simulink model "ibob_phased_array_2k"  (Simulink 7.0)
settings: Solver=ode45  StartTime=0.0  StopTime=70  RelTol=1e-3
undefined symbols (not defined in the file or in its folder): iBOB
libraries: xbsIndex_r4 x666, xps_library x63, beamform x4, casper_library x3
(part 2 of 6)

== system ibob_phased_array_2k/demux2 ==
  vin : Inport  OutDataType=sfix(16)  OutScaling=2^0
  in : Inport  Port=2  OutDataType=sfix(16)  OutScaling=2^0
  Counter : xbsIndex_r4/Counter  cnt_type=Free Running  cnt_to=Inf  operation=Up  start_count=0  cnt_by_val=1  arith_type=Unsigned  n_bits=1  bin_pt=0  load_pin=off  rst=off  en=on  explicit_period=off  period=1  dbl_ovrd=off  use_behavioral_HDL=off  use_rpm=on  implementation=Fabric  block_type=counter
      settings: xl_area=[0, 0, 0, 0, 0, 0, 0]
  Down Sample : xbsIndex_r4/Down Sample  sample_ratio=2  sample_phase=First Value of Frame  en=off  latency=1  dbl_ovrd=off  block_type=dsamp
      settings: xl_area=[0, 0, 0, 0, 0, 0, 0]  block_version=10.1.3
  Down Sample1 : xbsIndex_r4/Down Sample  sample_ratio=2  sample_phase="Last Value of Frame  (most efficient)"  en=off  latency=1  dbl_ovrd=off  block_type=dsamp
      settings: xl_area=[0, 0, 0, 0, 0, 0, 0]  block_version=10.1.3
  Slice1 : xbsIndex_r4/Slice  nbits=1  boolean_output=on  mode=Lower Bit Location + Width  bit1=0  base1=MSB of Input  bit0=0  base0=LSB of Input  dbl_ovrd=off  block_type=slice
      settings: infoedit="Extracts a given range of bits from each input sample and presents it at the output.  The output type is ordinarily unsigned with binary point at zero, but can be Boolean when the slice is one bit wide.<P><P>Hardware notes: In hardware this block costs nothing."  block_version=10.1.3
  out0 : Outport  OutDataType=sfix(16)  OutScaling=2^0
  out1 : Outport  Port=2  OutDataType=sfix(16)  OutScaling=2^0
  valid : Outport  Port=3  OutDataType=sfix(16)  OutScaling=2^0
  wires:
  in/1 -> Down Sample/1, Down Sample1/1
  Down Sample/1 -> out0/1
  Down Sample1/1 -> out1/1
  Counter/1 -> Slice1/1
  vin/1 -> Counter/1
  Slice1/1 -> valid/1

== system ibob_phased_array_2k/gain_calib0 ==
  gain : Inport  OutDataType=sfix(16)  OutScaling=2^0
  in : Inport  Port=2  OutDataType=sfix(16)  OutScaling=2^0
  Concat : xbsIndex_r4/Concat  num_inputs=4  dbl_ovrd=off  block_type=concat
      settings: block_version=10.1.3
  Convert{,1..3} (4 alike) : xbsIndex_r4/Convert  arith_type="Signed  (2's comp)"  n_bits=8  bin_pt=0  quantization=Truncate  overflow=Saturate  latency=0  dbl_ovrd=off  pipeline=off  block_type=convert
      settings: xl_area=[0, 0, 0, 0, 0, 0, 0]  block_version=10.1.3
  Convert4 : xbsIndex_r4/Convert  arith_type=Unsigned  n_bits=8  bin_pt=7  quantization=Truncate  overflow=Saturate  latency=0  dbl_ovrd=off  pipeline=off  block_type=convert
      settings: xl_area=[0, 0, 0, 0, 0, 0, 0]  block_version=10.1.3
  Mult{,1..3} (4 alike) : xbsIndex_r4/Mult  precision=Full  arith_type="Signed  (2's comp)"  n_bits=8  bin_pt=2  quantization=Truncate  overflow=Wrap  en=off  latency=5  dbl_ovrd=off  use_behavioral_HDL=off  use_embedded=on  opt=Speed  optimum_pipeline=off  pipeline=on  use_rpm=on  placement_style=Rectangular shape  block_type=mult
      settings: infoedit=Hardware notes: To use the internal pipeline stage of the dedicated multiplier you must select 'Pipeline for maximum performance'.  xl_area=[0, 0, 0, 0, 0, 0, 0]  block_version=10.1.3
  Reinterpret{,1..3} (4 alike) : xbsIndex_r4/Reinterpret  force_arith_type=on  arith_type=Unsigned  force_bin_pt=on  bin_pt=0  block_type=reinterpret
      settings: infoedit="Changes signal type without altering the binary representation.   You can changed the signal between signed and unsigned, and relocate the binary point.<P><P>Hardware notes: In hardware this block costs nothing.<P><P>Example:  Suppose the input is 6 bits wide, signed, with 2 fractional bits, and the output is forced to unsigned with 0 fractional bits.  Then an input of -2.0 (1110.00 in binary 2's complement) becomes an output of 56 (111000 in binary)."  block_version=10.1.3
  slice2 : Subsystem
  out : Outport  OutDataType=sfix(16)  OutScaling=2^0
  wires:
  in/1 -> slice2/1(in)
  slice2/1(out0) -> Mult/1
  slice2/2(out1) -> Mult1/1
  slice2/3(out2) -> Mult2/1
  slice2/4(out3) -> Mult3/1
  gain/1 -> Convert4/1
  Mult/1 -> Convert/1
  Mult1/1 -> Convert1/1
  Mult2/1 -> Convert2/1
  Mult3/1 -> Convert3/1
  Concat/1 -> out/1
  Convert3/1 -> Reinterpret3/1
  Convert2/1 -> Reinterpret2/1
  Convert1/1 -> Reinterpret1/1
  Convert/1 -> Reinterpret/1
  Convert4/1 -> Mult3/2, Mult2/2, Mult1/2, Mult/2
  Reinterpret/1 -> Concat/1
  Reinterpret1/1 -> Concat/2
  Reinterpret2/1 -> Concat/3
  Reinterpret3/1 -> Concat/4

== system ibob_phased_array_2k/gain_calib1 ==
  gain : Inport  OutDataType=sfix(16)  OutScaling=2^0
  in : Inport  Port=2  OutDataType=sfix(16)  OutScaling=2^0
  Concat : xbsIndex_r4/Concat  num_inputs=4  dbl_ovrd=off  block_type=concat
      settings: block_version=10.1.3
  Convert{,1..3} (4 alike) : xbsIndex_r4/Convert  arith_type="Signed  (2's comp)"  n_bits=8  bin_pt=0  quantization=Truncate  overflow=Saturate  latency=0  dbl_ovrd=off  pipeline=off  block_type=convert
      settings: xl_area=[0, 0, 0, 0, 0, 0, 0]  block_version=10.1.3
  Convert4 : xbsIndex_r4/Convert  arith_type=Unsigned  n_bits=8  bin_pt=7  quantization=Truncate  overflow=Saturate  latency=0  dbl_ovrd=off  pipeline=off  block_type=convert
      settings: xl_area=[0, 0, 0, 0, 0, 0, 0]  block_version=10.1.3
  Mult{,1..3} (4 alike) : xbsIndex_r4/Mult  precision=Full  arith_type="Signed  (2's comp)"  n_bits=8  bin_pt=2  quantization=Truncate  overflow=Wrap  en=off  latency=5  dbl_ovrd=off  use_behavioral_HDL=off  use_embedded=on  opt=Speed  optimum_pipeline=off  pipeline=on  use_rpm=on  placement_style=Rectangular shape  block_type=mult
      settings: infoedit=Hardware notes: To use the internal pipeline stage of the dedicated multiplier you must select 'Pipeline for maximum performance'.  xl_area=[0, 0, 0, 0, 0, 0, 0]  block_version=10.1.3
  Reinterpret{,1..3} (4 alike) : xbsIndex_r4/Reinterpret  force_arith_type=on  arith_type=Unsigned  force_bin_pt=on  bin_pt=0  block_type=reinterpret
      settings: infoedit="Changes signal type without altering the binary representation.   You can changed the signal between signed and unsigned, and relocate the binary point.<P><P>Hardware notes: In hardware this block costs nothing.<P><P>Example:  Suppose the input is 6 bits wide, signed, with 2 fractional bits, and the output is forced to unsigned with 0 fractional bits.  Then an input of -2.0 (1110.00 in binary 2's complement) becomes an output of 56 (111000 in binary)."  block_version=10.1.3
  slice2 : Subsystem
  out : Outport  OutDataType=sfix(16)  OutScaling=2^0
  wires:
  Reinterpret3/1 -> Concat/4
  Reinterpret2/1 -> Concat/3
  Reinterpret1/1 -> Concat/2
  Reinterpret/1 -> Concat/1
  Convert4/1 -> Mult/2, Mult1/2, Mult2/2, Mult3/2
  Convert/1 -> Reinterpret/1
  Convert1/1 -> Reinterpret1/1
  Convert2/1 -> Reinterpret2/1
  Convert3/1 -> Reinterpret3/1
  Concat/1 -> out/1
  Mult3/1 -> Convert3/1
  Mult2/1 -> Convert2/1
  Mult1/1 -> Convert1/1
  Mult/1 -> Convert/1
  gain/1 -> Convert4/1
  slice2/4(out3) -> Mult3/1
  slice2/3(out2) -> Mult2/1
  slice2/2(out1) -> Mult1/1
  slice2/1(out0) -> Mult/1
  in/1 -> slice2/1(in)

== system ibob_phased_array_2k/gain_calib2 ==
  gain : Inport  OutDataType=sfix(16)  OutScaling=2^0
  in : Inport  Port=2  OutDataType=sfix(16)  OutScaling=2^0
  Concat : xbsIndex_r4/Concat  num_inputs=4  dbl_ovrd=off  block_type=concat
      settings: block_version=10.1.3
  Convert{,1..3} (4 alike) : xbsIndex_r4/Convert  arith_type="Signed  (2's comp)"  n_bits=8  bin_pt=0  quantization=Truncate  overflow=Saturate  latency=0  dbl_ovrd=off  pipeline=off  block_type=convert
      settings: xl_area=[0, 0, 0, 0, 0, 0, 0]  block_version=10.1.3
  Convert4 : xbsIndex_r4/Convert  arith_type=Unsigned  n_bits=8  bin_pt=7  quantization=Truncate  overflow=Saturate  latency=0  dbl_ovrd=off  pipeline=off  block_type=convert
      settings: xl_area=[0, 0, 0, 0, 0, 0, 0]  block_version=10.1.3
  Mult{,1..3} (4 alike) : xbsIndex_r4/Mult  precision=Full  arith_type="Signed  (2's comp)"  n_bits=8  bin_pt=2  quantization=Truncate  overflow=Wrap  en=off  latency=5  dbl_ovrd=off  use_behavioral_HDL=off  use_embedded=on  opt=Speed  optimum_pipeline=off  pipeline=on  use_rpm=on  placement_style=Rectangular shape  block_type=mult
      settings: infoedit=Hardware notes: To use the internal pipeline stage of the dedicated multiplier you must select 'Pipeline for maximum performance'.  xl_area=[0, 0, 0, 0, 0, 0, 0]  block_version=10.1.3
  Reinterpret{,1..3} (4 alike) : xbsIndex_r4/Reinterpret  force_arith_type=on  arith_type=Unsigned  force_bin_pt=on  bin_pt=0  block_type=reinterpret
      settings: infoedit="Changes signal type without altering the binary representation.   You can changed the signal between signed and unsigned, and relocate the binary point.<P><P>Hardware notes: In hardware this block costs nothing.<P><P>Example:  Suppose the input is 6 bits wide, signed, with 2 fractional bits, and the output is forced to unsigned with 0 fractional bits.  Then an input of -2.0 (1110.00 in binary 2's complement) becomes an output of 56 (111000 in binary)."  block_version=10.1.3
  slice2 : Subsystem
  out : Outport  OutDataType=sfix(16)  OutScaling=2^0
  wires:
  Reinterpret3/1 -> Concat/4
  Reinterpret2/1 -> Concat/3
  Reinterpret1/1 -> Concat/2
  Reinterpret/1 -> Concat/1
  Convert4/1 -> Mult/2, Mult1/2, Mult2/2, Mult3/2
  Convert/1 -> Reinterpret/1
  Convert1/1 -> Reinterpret1/1
  Convert2/1 -> Reinterpret2/1
  Convert3/1 -> Reinterpret3/1
  Concat/1 -> out/1
  Mult3/1 -> Convert3/1
  Mult2/1 -> Convert2/1
  Mult1/1 -> Convert1/1
  Mult/1 -> Convert/1
  gain/1 -> Convert4/1
  slice2/4(out3) -> Mult3/1
  slice2/3(out2) -> Mult2/1
  slice2/2(out1) -> Mult1/1
  slice2/1(out0) -> Mult/1
  in/1 -> slice2/1(in)

== system ibob_phased_array_2k/gain_calib3 ==
  gain : Inport  OutDataType=sfix(16)  OutScaling=2^0
  in : Inport  Port=2  OutDataType=sfix(16)  OutScaling=2^0
  Concat : xbsIndex_r4/Concat  num_inputs=4  dbl_ovrd=off  block_type=concat
      settings: block_version=10.1.3
  Convert{,1..3} (4 alike) : xbsIndex_r4/Convert  arith_type="Signed  (2's comp)"  n_bits=8  bin_pt=0  quantization=Truncate  overflow=Saturate  latency=0  dbl_ovrd=off  pipeline=off  block_type=convert
      settings: xl_area=[0, 0, 0, 0, 0, 0, 0]  block_version=10.1.3
  Convert4 : xbsIndex_r4/Convert  arith_type=Unsigned  n_bits=8  bin_pt=7  quantization=Truncate  overflow=Saturate  latency=0  dbl_ovrd=off  pipeline=off  block_type=convert
      settings: xl_area=[0, 0, 0, 0, 0, 0, 0]  block_version=10.1.3
  Mult{,1..3} (4 alike) : xbsIndex_r4/Mult  precision=Full  arith_type="Signed  (2's comp)"  n_bits=8  bin_pt=2  quantization=Truncate  overflow=Wrap  en=off  latency=5  dbl_ovrd=off  use_behavioral_HDL=off  use_embedded=on  opt=Speed  optimum_pipeline=off  pipeline=on  use_rpm=on  placement_style=Rectangular shape  block_type=mult
      settings: infoedit=Hardware notes: To use the internal pipeline stage of the dedicated multiplier you must select 'Pipeline for maximum performance'.  xl_area=[0, 0, 0, 0, 0, 0, 0]  block_version=10.1.3
  Reinterpret{,1..3} (4 alike) : xbsIndex_r4/Reinterpret  force_arith_type=on  arith_type=Unsigned  force_bin_pt=on  bin_pt=0  block_type=reinterpret
      settings: infoedit="Changes signal type without altering the binary representation.   You can changed the signal between signed and unsigned, and relocate the binary point.<P><P>Hardware notes: In hardware this block costs nothing.<P><P>Example:  Suppose the input is 6 bits wide, signed, with 2 fractional bits, and the output is forced to unsigned with 0 fractional bits.  Then an input of -2.0 (1110.00 in binary 2's complement) becomes an output of 56 (111000 in binary)."  block_version=10.1.3
  slice2 : Subsystem
  out : Outport  OutDataType=sfix(16)  OutScaling=2^0
  wires:
  in/1 -> slice2/1(in)
  slice2/1(out0) -> Mult/1
  slice2/2(out1) -> Mult1/1
  slice2/3(out2) -> Mult2/1
  slice2/4(out3) -> Mult3/1
  gain/1 -> Convert4/1
  Mult/1 -> Convert/1
  Mult1/1 -> Convert1/1
  Mult2/1 -> Convert2/1
  Mult3/1 -> Convert3/1
  Concat/1 -> out/1
  Convert3/1 -> Reinterpret3/1
  Convert2/1 -> Reinterpret2/1
  Convert1/1 -> Reinterpret1/1
  Convert/1 -> Reinterpret/1
  Convert4/1 -> Mult3/2, Mult2/2, Mult1/2, Mult/2
  Reinterpret/1 -> Concat/1
  Reinterpret1/1 -> Concat/2
  Reinterpret2/1 -> Concat/3
  Reinterpret3/1 -> Concat/4

== system ibob_phased_array_2k/latch ==
  sw : Inport  OutDataType=sfix(16)  OutScaling=2^0
  rst : Inport  Port=2  OutDataType=sfix(16)  OutScaling=2^0
  1bit_count : xbsIndex_r4/Counter  cnt_type=Free Running  cnt_to=Inf  operation=Up  start_count=0  cnt_by_val=1  arith_type=Unsigned  n_bits=1  bin_pt=0  load_pin=off  rst=on  en=on  explicit_period=off  period=1  dbl_ovrd=off  use_behavioral_HDL=off  use_rpm=on  implementation=Fabric  block_type=counter
      settings: xl_area=[0, 0, 0, 0, 0, 0, 0]
  Convert1 : xbsIndex_r4/Convert  Orientation=left  arith_type=Boolean  n_bits=1  bin_pt=0  quantization=Truncate  overflow=Wrap  latency=0  dbl_ovrd=off  pipeline=off  block_type=convert
      settings: xl_area=[0, 0, 0, 0, 0, 0, 0]  block_version=10.1.3
  Convert2 : xbsIndex_r4/Convert  arith_type=Boolean  n_bits=1  bin_pt=0  quantization=Truncate  overflow=Wrap  latency=0  dbl_ovrd=off  pipeline=off  block_type=convert
      settings: xl_area=[0, 0, 0, 0, 0, 0, 0]  block_version=10.1.3
  Inverter : xbsIndex_r4/Inverter  Orientation=left  en=off  latency=0  dbl_ovrd=off  block_type=inv
      settings: xl_area=[0, 0, 0, 0, 0, 0, 0]
  Logical : xbsIndex_r4/Logical  logical_function=AND  inputs=2  en=off  latency=0  precision=Full  arith_type=Unsigned  n_bits=8  bin_pt=2  align_bp=on  dbl_ovrd=off  block_type=logical
      settings: xl_area=[0, 0, 0, 0, 0, 0, 0]
  out : Outport  OutDataType=sfix(16)  OutScaling=2^0
  wires:
  1bit_count/1 -> Inverter/1, Convert2/1
  rst/1 -> 1bit_count/1
  Convert2/1 -> out/1
  Logical/1 -> 1bit_count/2
  sw/1 -> Logical/1
  Inverter/1 -> Convert1/1
  Convert1/1 -> Logical/2

== system ibob_phased_array_2k/quant0 ==
  thresh : Inport  Orientation=down  OutDataType=sfix(16)  OutScaling=2^0
  walsh : Inport  Orientation=down  Port=2  OutDataType=sfix(16)  OutScaling=2^0
  in0 : Inport  Port=3  OutDataType=sfix(16)  OutScaling=2^0
  in1 : Inport  Port=4  OutDataType=sfix(16)  OutScaling=2^0
  in2 : Inport  Port=5  OutDataType=sfix(16)  OutScaling=2^0
  in3 : Inport  Port=6  OutDataType=sfix(16)  OutScaling=2^0
  2bit_quantizer_0 : Subsystem
  2bit_quantizer_1 : Subsystem
  2bit_quantizer_2 : Subsystem
  2bit_quantizer_3 : Subsystem
  Concat1 : xbsIndex_r4/Concat  num_inputs=4  dbl_ovrd=off  block_type=concat
      settings: block_version=10.1.3
  Concat2 : xbsIndex_r4/Concat  num_inputs=4  dbl_ovrd=off  block_type=concat
      settings: block_version=10.1.3
  cat_out : Outport  OutDataType=sfix(16)  OutScaling=2^0
  8bit_out : Outport  Port=2  OutDataType=sfix(16)  OutScaling=2^0
  wires:
  thresh/1 -> 2bit_quantizer_0/2(thresh), 2bit_quantizer_2/2(thresh), 2bit_quantizer_3/2(thresh), 2bit_quantizer_1/2(thresh)
  2bit_quantizer_0/1(out) -> Concat1/1
  2bit_quantizer_1/1(out) -> Concat1/2
  2bit_quantizer_2/1(out) -> Concat1/3
  2bit_quantizer_3/1(out) -> Concat1/4
  in0/1 -> 2bit_quantizer_0/1(in)
  in1/1 -> 2bit_quantizer_1/1(in)
  Concat1/1 -> cat_out/1
  in2/1 -> 2bit_quantizer_2/1(in)
  in3/1 -> 2bit_quantizer_3/1(in)
  walsh/1 -> 2bit_quantizer_2/3(walsh), 2bit_quantizer_3/3(walsh), 2bit_quantizer_1/3(walsh), 2bit_quantizer_0/3(walsh)
  Concat2/1 -> 8bit_out/1
  2bit_quantizer_0/2(8bit_out) -> Concat2/1
  2bit_quantizer_1/2(8bit_out) -> Concat2/2
  2bit_quantizer_2/2(8bit_out) -> Concat2/3
  2bit_quantizer_3/2(8bit_out) -> Concat2/4

== system ibob_phased_array_2k/quant1 ==
  thresh : Inport  Orientation=down  OutDataType=sfix(16)  OutScaling=2^0
  walsh : Inport  Orientation=down  Port=2  OutDataType=sfix(16)  OutScaling=2^0
  in0 : Inport  Port=3  OutDataType=sfix(16)  OutScaling=2^0
  in1 : Inport  Port=4  OutDataType=sfix(16)  OutScaling=2^0
  in2 : Inport  Port=5  OutDataType=sfix(16)  OutScaling=2^0
  in3 : Inport  Port=6  OutDataType=sfix(16)  OutScaling=2^0
  2bit_quantizer_0 : Subsystem
  2bit_quantizer_1 : Subsystem
  2bit_quantizer_2 : Subsystem
  2bit_quantizer_3 : Subsystem
  Concat1 : xbsIndex_r4/Concat  num_inputs=4  dbl_ovrd=off  block_type=concat
      settings: block_version=10.1.3
  Concat2 : xbsIndex_r4/Concat  num_inputs=4  dbl_ovrd=off  block_type=concat
      settings: block_version=10.1.3
  cat_out : Outport  OutDataType=sfix(16)  OutScaling=2^0
  8bit_out : Outport  Port=2  OutDataType=sfix(16)  OutScaling=2^0
  wires:
  2bit_quantizer_3/2(8bit_out) -> Concat2/4
  2bit_quantizer_2/2(8bit_out) -> Concat2/3
  2bit_quantizer_1/2(8bit_out) -> Concat2/2
  2bit_quantizer_0/2(8bit_out) -> Concat2/1
  Concat2/1 -> 8bit_out/1
  walsh/1 -> 2bit_quantizer_0/3(walsh), 2bit_quantizer_1/3(walsh), 2bit_quantizer_3/3(walsh), 2bit_quantizer_2/3(walsh)
  in3/1 -> 2bit_quantizer_3/1(in)
  in2/1 -> 2bit_quantizer_2/1(in)
  Concat1/1 -> cat_out/1
  in1/1 -> 2bit_quantizer_1/1(in)
  in0/1 -> 2bit_quantizer_0/1(in)
  2bit_quantizer_3/1(out) -> Concat1/4
  2bit_quantizer_2/1(out) -> Concat1/3
  2bit_quantizer_1/1(out) -> Concat1/2
  2bit_quantizer_0/1(out) -> Concat1/1
  thresh/1 -> 2bit_quantizer_1/2(thresh), 2bit_quantizer_3/2(thresh), 2bit_quantizer_2/2(thresh), 2bit_quantizer_0/2(thresh)

== system ibob_phased_array_2k/quant2 ==
  thresh : Inport  Orientation=down  OutDataType=sfix(16)  OutScaling=2^0
  walsh : Inport  Orientation=down  Port=2  OutDataType=sfix(16)  OutScaling=2^0
  in0 : Inport  Port=3  OutDataType=sfix(16)  OutScaling=2^0
  in1 : Inport  Port=4  OutDataType=sfix(16)  OutScaling=2^0
  in2 : Inport  Port=5  OutDataType=sfix(16)  OutScaling=2^0
  in3 : Inport  Port=6  OutDataType=sfix(16)  OutScaling=2^0
  2bit_quantizer_0 : Subsystem
  2bit_quantizer_1 : Subsystem
  2bit_quantizer_2 : Subsystem
  2bit_quantizer_3 : Subsystem
  Concat1 : xbsIndex_r4/Concat  num_inputs=4  dbl_ovrd=off  block_type=concat
      settings: block_version=10.1.3
  Concat2 : xbsIndex_r4/Concat  num_inputs=4  dbl_ovrd=off  block_type=concat
      settings: block_version=10.1.3
  cat_out : Outport  OutDataType=sfix(16)  OutScaling=2^0
  8bit_out : Outport  Port=2  OutDataType=sfix(16)  OutScaling=2^0
  wires:
  thresh/1 -> 2bit_quantizer_0/2(thresh), 2bit_quantizer_2/2(thresh), 2bit_quantizer_3/2(thresh), 2bit_quantizer_1/2(thresh)
  2bit_quantizer_0/1(out) -> Concat1/1
  2bit_quantizer_1/1(out) -> Concat1/2
  2bit_quantizer_2/1(out) -> Concat1/3
  2bit_quantizer_3/1(out) -> Concat1/4
  in0/1 -> 2bit_quantizer_0/1(in)
  in1/1 -> 2bit_quantizer_1/1(in)
  Concat1/1 -> cat_out/1
  in2/1 -> 2bit_quantizer_2/1(in)
  in3/1 -> 2bit_quantizer_3/1(in)
  walsh/1 -> 2bit_quantizer_2/3(walsh), 2bit_quantizer_3/3(walsh), 2bit_quantizer_1/3(walsh), 2bit_quantizer_0/3(walsh)
  Concat2/1 -> 8bit_out/1
  2bit_quantizer_0/2(8bit_out) -> Concat2/1
  2bit_quantizer_1/2(8bit_out) -> Concat2/2
  2bit_quantizer_2/2(8bit_out) -> Concat2/3
  2bit_quantizer_3/2(8bit_out) -> Concat2/4

== system ibob_phased_array_2k/quant3 ==
  thresh : Inport  Orientation=down  OutDataType=sfix(16)  OutScaling=2^0
  walsh : Inport  Orientation=down  Port=2  OutDataType=sfix(16)  OutScaling=2^0
  in0 : Inport  Port=3  OutDataType=sfix(16)  OutScaling=2^0
  in1 : Inport  Port=4  OutDataType=sfix(16)  OutScaling=2^0
  in2 : Inport  Port=5  OutDataType=sfix(16)  OutScaling=2^0
  in3 : Inport  Port=6  OutDataType=sfix(16)  OutScaling=2^0
  2bit_quantizer_0 : Subsystem
  2bit_quantizer_1 : Subsystem
  2bit_quantizer_2 : Subsystem
  2bit_quantizer_3 : Subsystem
  Concat1 : xbsIndex_r4/Concat  num_inputs=4  dbl_ovrd=off  block_type=concat
      settings: block_version=10.1.3
  Concat2 : xbsIndex_r4/Concat  num_inputs=4  dbl_ovrd=off  block_type=concat
      settings: block_version=10.1.3
  cat_out : Outport  OutDataType=sfix(16)  OutScaling=2^0
  8bit_out : Outport  Port=2  OutDataType=sfix(16)  OutScaling=2^0
  wires:
  2bit_quantizer_3/2(8bit_out) -> Concat2/4
  2bit_quantizer_2/2(8bit_out) -> Concat2/3
  2bit_quantizer_1/2(8bit_out) -> Concat2/2
  2bit_quantizer_0/2(8bit_out) -> Concat2/1
  Concat2/1 -> 8bit_out/1
  walsh/1 -> 2bit_quantizer_0/3(walsh), 2bit_quantizer_1/3(walsh), 2bit_quantizer_3/3(walsh), 2bit_quantizer_2/3(walsh)
  in3/1 -> 2bit_quantizer_3/1(in)
  in2/1 -> 2bit_quantizer_2/1(in)
  Concat1/1 -> cat_out/1
  in1/1 -> 2bit_quantizer_1/1(in)
  in0/1 -> 2bit_quantizer_0/1(in)
  2bit_quantizer_3/1(out) -> Concat1/4
  2bit_quantizer_2/1(out) -> Concat1/3
  2bit_quantizer_1/1(out) -> Concat1/2
  2bit_quantizer_0/1(out) -> Concat1/1
  thresh/1 -> 2bit_quantizer_1/2(thresh), 2bit_quantizer_3/2(thresh), 2bit_quantizer_2/2(thresh), 2bit_quantizer_0/2(thresh)

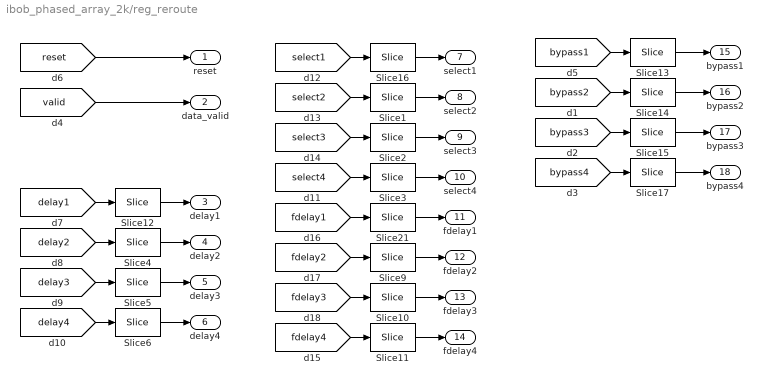
== system ibob_phased_array_2k/reg_reroute ==
  Slice{1..3,16} (4 alike) : xbsIndex_r4/Slice  nbits=1  boolean_output=off  mode=Two Bit Locations  bit1=1  base1=LSB of Input  bit0=0  base0=LSB of Input  dbl_ovrd=off  block_type=slice
      settings: infoedit="Extracts a given range of bits from each input sample and presents it at the output.  The output type is ordinarily unsigned with binary point at zero, but can be Boolean when the slice is one bit wide.<P><P>Hardware notes: In hardware this block costs nothing."  block_version=10.1.3
  Slice{9..11,21} (4 alike) : xbsIndex_r4/Slice  nbits=1  boolean_output=off  mode=Two Bit Locations  bit1=3  base1=LSB of Input  bit0=0  base0=LSB of Input  dbl_ovrd=off  block_type=slice
      settings: infoedit="Extracts a given range of bits from each input sample and presents it at the output.  The output type is ordinarily unsigned with binary point at zero, but can be Boolean when the slice is one bit wide.<P><P>Hardware notes: In hardware this block costs nothing."  block_version=10.1.3
  Slice{4..6,12} (4 alike) : xbsIndex_r4/Slice  nbits=1  boolean_output=off  mode=Two Bit Locations  bit1=10  base1=LSB of Input  bit0=0  base0=LSB of Input  dbl_ovrd=off  block_type=slice
      settings: infoedit="Extracts a given range of bits from each input sample and presents it at the output.  The output type is ordinarily unsigned with binary point at zero, but can be Boolean when the slice is one bit wide.<P><P>Hardware notes: In hardware this block costs nothing."  block_version=10.1.3
  Slice{13..15,17} (4 alike) : xbsIndex_r4/Slice  nbits=1  boolean_output=on  mode=Lower Bit Location + Width  bit1=9  base1=LSB of Input  bit0=0  base0=LSB of Input  dbl_ovrd=off  block_type=slice
      settings: infoedit="Extracts a given range of bits from each input sample and presents it at the output.  The output type is ordinarily unsigned with binary point at zero, but can be Boolean when the slice is one bit wide.<P><P>Hardware notes: In hardware this block costs nothing."  block_version=10.1.3
  reset : Outport  OutDataType=sfix(16)  OutScaling=2^0
  data_valid : Outport  Port=2  OutDataType=sfix(16)  OutScaling=2^0
  delay1 : Outport  Port=3  OutDataType=sfix(16)  OutScaling=2^0
  delay2 : Outport  Port=4  OutDataType=sfix(16)  OutScaling=2^0
  delay3 : Outport  Port=5  OutDataType=sfix(16)  OutScaling=2^0
  delay4 : Outport  Port=6  OutDataType=sfix(16)  OutScaling=2^0
  select1 : Outport  Port=7  OutDataType=sfix(16)  OutScaling=2^0
  select2 : Outport  Port=8  OutDataType=sfix(16)  OutScaling=2^0
  select3 : Outport  Port=9  OutDataType=sfix(16)  OutScaling=2^0
  select4 : Outport  Port=10  OutDataType=sfix(16)  OutScaling=2^0
  fdelay1 : Outport  Port=11  OutDataType=sfix(16)  OutScaling=2^0
  fdelay2 : Outport  Port=12  OutDataType=sfix(16)  OutScaling=2^0
  fdelay3 : Outport  Port=13  OutDataType=sfix(16)  OutScaling=2^0
  fdelay4 : Outport  Port=14  OutDataType=sfix(16)  OutScaling=2^0
  bypass1 : Outport  Port=15  OutDataType=sfix(16)  OutScaling=2^0
  bypass2 : Outport  Port=16  OutDataType=sfix(16)  OutScaling=2^0
  bypass3 : Outport  Port=17  OutDataType=sfix(16)  OutScaling=2^0
  bypass4 : Outport  Port=18  OutDataType=sfix(16)  OutScaling=2^0
  wires:
  [valid] -> data_valid/1
  [bypass1] -> Slice13/1
  [reset] -> reset/1
  [delay1] -> Slice12/1
  [delay2] -> Slice4/1
  [delay3] -> Slice5/1
  [delay4] -> Slice6/1
  [select4] -> Slice3/1
  [select3] -> Slice2/1
  [select2] -> Slice1/1
  [select1] -> Slice16/1
  [fdelay4] -> Slice11/1
  [fdelay3] -> Slice10/1
  [fdelay2] -> Slice9/1
  [fdelay1] -> Slice21/1
  [bypass2] -> Slice14/1
  [bypass3] -> Slice15/1
  [bypass4] -> Slice17/1
  Slice16/1 -> select1/1
  Slice1/1 -> select2/1
  Slice2/1 -> select3/1
  Slice3/1 -> select4/1
  Slice12/1 -> delay1/1
  Slice4/1 -> delay2/1
  Slice5/1 -> delay3/1
  Slice6/1 -> delay4/1
  Slice21/1 -> fdelay1/1
  Slice9/1 -> fdelay2/1
  Slice10/1 -> fdelay3/1
  Slice11/1 -> fdelay4/1
  Slice13/1 -> bypass1/1
  Slice14/1 -> bypass2/1
  Slice15/1 -> bypass3/1
  Slice17/1 -> bypass4/1

== system ibob_phased_array_2k/slice0 ==
  in : Inport  OutDataType=sfix(16)  OutScaling=2^0
  Slice1 : xbsIndex_r4/Slice  nbits=8  boolean_output=off  mode=Upper Bit Location + Width  bit1=-16  base1=MSB of Input  bit0=0  base0=LSB of Input  dbl_ovrd=off  block_type=slice
      settings: infoedit="Extracts a given range of bits from each input sample and presents it at the output.  The output type is ordinarily unsigned with binary point at zero, but can be Boolean when the slice is one bit wide.<P><P>Hardware notes: In hardware this block costs nothing."  block_version=10.1.3
  Slice2 : xbsIndex_r4/Slice  nbits=8  boolean_output=off  mode=Upper Bit Location + Width  bit1=-24  base1=MSB of Input  bit0=0  base0=LSB of Input  dbl_ovrd=off  block_type=slice
      settings: infoedit="Extracts a given range of bits from each input sample and presents it at the output.  The output type is ordinarily unsigned with binary point at zero, but can be Boolean when the slice is one bit wide.<P><P>Hardware notes: In hardware this block costs nothing."  block_version=10.1.3
  Slice26 : xbsIndex_r4/Slice  nbits=8  boolean_output=off  mode=Upper Bit Location + Width  bit1=0  base1=MSB of Input  bit0=0  base0=LSB of Input  dbl_ovrd=off  block_type=slice
      settings: infoedit="Extracts a given range of bits from each input sample and presents it at the output.  The output type is ordinarily unsigned with binary point at zero, but can be Boolean when the slice is one bit wide.<P><P>Hardware notes: In hardware this block costs nothing."  block_version=10.1.3
  Slice27 : xbsIndex_r4/Slice  nbits=8  boolean_output=off  mode=Upper Bit Location + Width  bit1=-8  base1=MSB of Input  bit0=0  base0=LSB of Input  dbl_ovrd=off  block_type=slice
      settings: infoedit="Extracts a given range of bits from each input sample and presents it at the output.  The output type is ordinarily unsigned with binary point at zero, but can be Boolean when the slice is one bit wide.<P><P>Hardware notes: In hardware this block costs nothing."  block_version=10.1.3
  out0 : Outport  OutDataType=sfix(16)  OutScaling=2^0
  out1 : Outport  Port=2  OutDataType=sfix(16)  OutScaling=2^0
  out2 : Outport  Port=3  OutDataType=sfix(16)  OutScaling=2^0
  out3 : Outport  Port=4  OutDataType=sfix(16)  OutScaling=2^0
  wires:
  in/1 -> Slice26/1, Slice27/1, Slice1/1, Slice2/1
  Slice26/1 -> out0/1
  Slice27/1 -> out1/1
  Slice1/1 -> out2/1
  Slice2/1 -> out3/1

== system ibob_phased_array_2k/slice1 ==
  in : Inport  OutDataType=sfix(16)  OutScaling=2^0
  Slice1 : xbsIndex_r4/Slice  nbits=8  boolean_output=off  mode=Upper Bit Location + Width  bit1=-16  base1=MSB of Input  bit0=0  base0=LSB of Input  dbl_ovrd=off  block_type=slice
      settings: infoedit="Extracts a given range of bits from each input sample and presents it at the output.  The output type is ordinarily unsigned with binary point at zero, but can be Boolean when the slice is one bit wide.<P><P>Hardware notes: In hardware this block costs nothing."  block_version=10.1.3
  Slice2 : xbsIndex_r4/Slice  nbits=8  boolean_output=off  mode=Upper Bit Location + Width  bit1=-24  base1=MSB of Input  bit0=0  base0=LSB of Input  dbl_ovrd=off  block_type=slice
      settings: infoedit="Extracts a given range of bits from each input sample and presents it at the output.  The output type is ordinarily unsigned with binary point at zero, but can be Boolean when the slice is one bit wide.<P><P>Hardware notes: In hardware this block costs nothing."  block_version=10.1.3
  Slice26 : xbsIndex_r4/Slice  nbits=8  boolean_output=off  mode=Upper Bit Location + Width  bit1=0  base1=MSB of Input  bit0=0  base0=LSB of Input  dbl_ovrd=off  block_type=slice
      settings: infoedit="Extracts a given range of bits from each input sample and presents it at the output.  The output type is ordinarily unsigned with binary point at zero, but can be Boolean when the slice is one bit wide.<P><P>Hardware notes: In hardware this block costs nothing."  block_version=10.1.3
  Slice27 : xbsIndex_r4/Slice  nbits=8  boolean_output=off  mode=Upper Bit Location + Width  bit1=-8  base1=MSB of Input  bit0=0  base0=LSB of Input  dbl_ovrd=off  block_type=slice
      settings: infoedit="Extracts a given range of bits from each input sample and presents it at the output.  The output type is ordinarily unsigned with binary point at zero, but can be Boolean when the slice is one bit wide.<P><P>Hardware notes: In hardware this block costs nothing."  block_version=10.1.3
  out0 : Outport  OutDataType=sfix(16)  OutScaling=2^0
  out1 : Outport  Port=2  OutDataType=sfix(16)  OutScaling=2^0
  out2 : Outport  Port=3  OutDataType=sfix(16)  OutScaling=2^0
  out3 : Outport  Port=4  OutDataType=sfix(16)  OutScaling=2^0
  wires:
  Slice2/1 -> out3/1
  Slice1/1 -> out2/1
  Slice27/1 -> out1/1
  Slice26/1 -> out0/1
  in/1 -> Slice2/1, Slice1/1, Slice27/1, Slice26/1

== system ibob_phased_array_2k/slice2 ==
  in : Inport  OutDataType=sfix(16)  OutScaling=2^0
  Slice1 : xbsIndex_r4/Slice  nbits=8  boolean_output=off  mode=Upper Bit Location + Width  bit1=-16  base1=MSB of Input  bit0=0  base0=LSB of Input  dbl_ovrd=off  block_type=slice
      settings: infoedit="Extracts a given range of bits from each input sample and presents it at the output.  The output type is ordinarily unsigned with binary point at zero, but can be Boolean when the slice is one bit wide.<P><P>Hardware notes: In hardware this block costs nothing."  block_version=10.1.3
  Slice2 : xbsIndex_r4/Slice  nbits=8  boolean_output=off  mode=Upper Bit Location + Width  bit1=-24  base1=MSB of Input  bit0=0  base0=LSB of Input  dbl_ovrd=off  block_type=slice
      settings: infoedit="Extracts a given range of bits from each input sample and presents it at the output.  The output type is ordinarily unsigned with binary point at zero, but can be Boolean when the slice is one bit wide.<P><P>Hardware notes: In hardware this block costs nothing."  block_version=10.1.3
  Slice26 : xbsIndex_r4/Slice  nbits=8  boolean_output=off  mode=Upper Bit Location + Width  bit1=0  base1=MSB of Input  bit0=0  base0=LSB of Input  dbl_ovrd=off  block_type=slice
      settings: infoedit="Extracts a given range of bits from each input sample and presents it at the output.  The output type is ordinarily unsigned with binary point at zero, but can be Boolean when the slice is one bit wide.<P><P>Hardware notes: In hardware this block costs nothing."  block_version=10.1.3
  Slice27 : xbsIndex_r4/Slice  nbits=8  boolean_output=off  mode=Upper Bit Location + Width  bit1=-8  base1=MSB of Input  bit0=0  base0=LSB of Input  dbl_ovrd=off  block_type=slice
      settings: infoedit="Extracts a given range of bits from each input sample and presents it at the output.  The output type is ordinarily unsigned with binary point at zero, but can be Boolean when the slice is one bit wide.<P><P>Hardware notes: In hardware this block costs nothing."  block_version=10.1.3
  out0 : Outport  OutDataType=sfix(16)  OutScaling=2^0
  out1 : Outport  Port=2  OutDataType=sfix(16)  OutScaling=2^0
  out2 : Outport  Port=3  OutDataType=sfix(16)  OutScaling=2^0
  out3 : Outport  Port=4  OutDataType=sfix(16)  OutScaling=2^0
  wires:
  in/1 -> Slice26/1, Slice27/1, Slice1/1, Slice2/1
  Slice26/1 -> out0/1
  Slice27/1 -> out1/1
  Slice1/1 -> out2/1
  Slice2/1 -> out3/1

== system ibob_phased_array_2k/slice3 ==
  in : Inport  OutDataType=sfix(16)  OutScaling=2^0
  Slice1 : xbsIndex_r4/Slice  nbits=8  boolean_output=off  mode=Upper Bit Location + Width  bit1=-16  base1=MSB of Input  bit0=0  base0=LSB of Input  dbl_ovrd=off  block_type=slice
      settings: infoedit="Extracts a given range of bits from each input sample and presents it at the output.  The output type is ordinarily unsigned with binary point at zero, but can be Boolean when the slice is one bit wide.<P><P>Hardware notes: In hardware this block costs nothing."  block_version=10.1.3
  Slice2 : xbsIndex_r4/Slice  nbits=8  boolean_output=off  mode=Upper Bit Location + Width  bit1=-24  base1=MSB of Input  bit0=0  base0=LSB of Input  dbl_ovrd=off  block_type=slice
      settings: infoedit="Extracts a given range of bits from each input sample and presents it at the output.  The output type is ordinarily unsigned with binary point at zero, but can be Boolean when the slice is one bit wide.<P><P>Hardware notes: In hardware this block costs nothing."  block_version=10.1.3
  Slice26 : xbsIndex_r4/Slice  nbits=8  boolean_output=off  mode=Upper Bit Location + Width  bit1=0  base1=MSB of Input  bit0=0  base0=LSB of Input  dbl_ovrd=off  block_type=slice
      settings: infoedit="Extracts a given range of bits from each input sample and presents it at the output.  The output type is ordinarily unsigned with binary point at zero, but can be Boolean when the slice is one bit wide.<P><P>Hardware notes: In hardware this block costs nothing."  block_version=10.1.3
  Slice27 : xbsIndex_r4/Slice  nbits=8  boolean_output=off  mode=Upper Bit Location + Width  bit1=-8  base1=MSB of Input  bit0=0  base0=LSB of Input  dbl_ovrd=off  block_type=slice
      settings: infoedit="Extracts a given range of bits from each input sample and presents it at the output.  The output type is ordinarily unsigned with binary point at zero, but can be Boolean when the slice is one bit wide.<P><P>Hardware notes: In hardware this block costs nothing."  block_version=10.1.3
  out0 : Outport  OutDataType=sfix(16)  OutScaling=2^0
  out1 : Outport  Port=2  OutDataType=sfix(16)  OutScaling=2^0
  out2 : Outport  Port=3  OutDataType=sfix(16)  OutScaling=2^0
  out3 : Outport  Port=4  OutDataType=sfix(16)  OutScaling=2^0
  wires:
  Slice2/1 -> out3/1
  Slice1/1 -> out2/1
  Slice27/1 -> out1/1
  Slice26/1 -> out0/1
  in/1 -> Slice2/1, Slice1/1, Slice27/1, Slice26/1

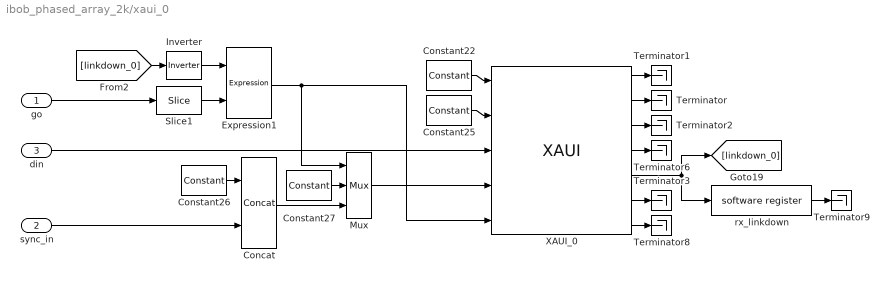
== system ibob_phased_array_2k/xaui_0 ==
  go : Inport  OutDataType=sfix(16)  OutScaling=2^0
  sync_in : Inport  Port=2  OutDataType=sfix(16)  OutScaling=2^0
  din : Inport  Port=3  OutDataType=sfix(16)  OutScaling=2^0
  Concat : xbsIndex_r4/Concat  num_inputs=2  dbl_ovrd=off  block_type=concat
      settings: block_version=10.1.3
  Constant22 : xbsIndex_r4/Constant  arith_type=Boolean  const=0  n_bits=32  bin_pt=0  explicit_period=on  period=1  equ=P=C  opselect=C  inp2=PCIN>>17  opr=+  inp1=P  carry=CIN  dbl_ovrd=off  block_type=constant
  Constant25 : xbsIndex_r4/Constant  arith_type=Boolean  const=0  n_bits=32  bin_pt=0  explicit_period=on  period=1  equ=P=C  opselect=C  inp2=PCIN>>17  opr=+  inp1=P  carry=CIN  dbl_ovrd=off  block_type=constant
  Constant26 : xbsIndex_r4/Constant  arith_type=Unsigned  const=0  n_bits=3  bin_pt=0  explicit_period=on  period=1  equ=P=C  opselect=C  inp2=PCIN>>17  opr=+  inp1=P  carry=CIN  dbl_ovrd=off  block_type=constant
  Constant27 : xbsIndex_r4/Constant  arith_type=Unsigned  const=0  n_bits=4  bin_pt=0  explicit_period=on  period=1  equ=P=C  opselect=C  inp2=PCIN>>17  opr=+  inp1=P  carry=CIN  dbl_ovrd=off  block_type=constant
  Expression1 : xbsIndex_r4/Expression  expression=a & b  align_bp=on  en=off  latency=0  precision=Full  arith_type=Unsigned  n_bits=8  bin_pt=2  dbl_ovrd=off  block_type=expr
      settings: xl_area=[0, 0, 0, 0, 0, 0, 0]  block_version=10.1.3
  Inverter : xbsIndex_r4/Inverter  en=off  latency=0  dbl_ovrd=off  block_type=inv
      settings: xl_area=[0, 0, 0, 0, 0, 0, 0]
  Mux : xbsIndex_r4/Mux  inputs=2  en=off  latency=0  precision=Full  arith_type="Signed  (2's comp)"  n_bits=8  bin_pt=2  quantization=Truncate  overflow=Wrap  dbl_ovrd=off  block_type=mux
      settings: xl_area=[0, 0, 0, 0, 0, 0, 0]
  Slice1 : xbsIndex_r4/Slice  nbits=1  boolean_output=on  mode=Lower Bit Location + Width  bit1=0  base1=MSB of Input  bit0=0  base0=LSB of Input  dbl_ovrd=off  block_type=slice
      settings: infoedit="Extracts a given range of bits from each input sample and presents it at the output.  The output type is ordinarily unsigned with binary point at zero, but can be Boolean when the slice is one bit wide.<P><P>Hardware notes: In hardware this block costs nothing."  block_version=10.1.3
  Terminator{,1..3,6,8..9} (7 alike) : Terminator
  XAUI_0 : xps_library/XAUI  Tag=xps:xaui  SystemSampleTime=-1  demux=2  port=iBOB:0  open_phy=off  show_param=off  pre_emph=3  swing=800
      link override convert_tx_data: n_bits=32
      link override convert_tx_outofband: n_bits=4
      link override ibob_phased_array_2k_xaui_0_XAUI_0_rx_data: n_bits=32
      link override ibob_phased_array_2k_xaui_0_XAUI_0_rx_outofband: n_bits=4
  rx_linkdown : xps_library/software register  Tag=xps:sw_reg  SystemSampleTime=-1  io_dir=To Processor  arith_type=Unsigned  bitwidth=32  bin_pt=0  sample_period=1  gw_name=ibob_phased_array_2k_xaui_0_rx_linkdown_user_data_in
      link override convert: arith_type=Unsigned  n_bits=32  bin_pt=0
  wires:
  XAUI_0/1 -> Terminator1/1
  XAUI_0/2 -> Terminator/1
  XAUI_0/3 -> Terminator2/1
  XAUI_0/4 -> Terminator6/1
  XAUI_0/5 -> [linkdown_0], rx_linkdown/1
  XAUI_0/7 -> Terminator8/1
  rx_linkdown/1 -> Terminator9/1
  Constant22/1 -> XAUI_0/1
  Constant25/1 -> XAUI_0/2
  [linkdown_0] -> Inverter/1
  Inverter/1 -> Expression1/1
  Slice1/1 -> Expression1/2
  Constant26/1 -> Concat/1
  sync_in/1 -> Concat/2
  Concat/1 -> Mux/3
  Constant27/1 -> Mux/2
  Mux/1 -> XAUI_0/4
  Expression1/1 -> Mux/1, XAUI_0/5
  din/1 -> XAUI_0/3
  go/1 -> Slice1/1
  XAUI_0/6 -> Terminator3/1

== system ibob_phased_array_2k/xaui_1 ==
  go : Inport  OutDataType=sfix(16)  OutScaling=2^0
  sync_in : Inport  Port=2  OutDataType=sfix(16)  OutScaling=2^0
  din : Inport  Port=3  OutDataType=sfix(16)  OutScaling=2^0
  Constant22 : xbsIndex_r4/Constant  arith_type=Boolean  const=0  n_bits=32  bin_pt=0  explicit_period=on  period=1  equ=P=C  opselect=C  inp2=PCIN>>17  opr=+  inp1=P  carry=CIN  dbl_ovrd=off  block_type=constant
  Constant25 : xbsIndex_r4/Constant  arith_type=Boolean  const=0  n_bits=32  bin_pt=0  explicit_period=on  period=1  equ=P=C  opselect=C  inp2=PCIN>>17  opr=+  inp1=P  carry=CIN  dbl_ovrd=off  block_type=constant
  Expression1 : xbsIndex_r4/Expression  expression=a & b  align_bp=on  en=off  latency=0  precision=Full  arith_type=Unsigned  n_bits=8  bin_pt=2  dbl_ovrd=off  block_type=expr
      settings: xl_area=[0, 0, 0, 0, 0, 0, 0]  block_version=10.1.3
  Inverter : xbsIndex_r4/Inverter  en=off  latency=0  dbl_ovrd=off  block_type=inv
      settings: xl_area=[0, 0, 0, 0, 0, 0, 0]
  Terminator{,1..3,6,8..9} (7 alike) : Terminator
  XAUI_1 : xps_library/XAUI  Tag=xps:xaui  SystemSampleTime=-1  demux=1  port=iBOB:1  open_phy=off  show_param=off  pre_emph=3  swing=800
      link override convert_tx_data: n_bits=64
      link override convert_tx_outofband: n_bits=8
      link override ibob_phased_array_2k_xaui_1_XAUI_1_rx_data: n_bits=64
      link override ibob_phased_array_2k_xaui_1_XAUI_1_rx_outofband: n_bits=8
  rx_linkdown : xps_library/software register  Tag=xps:sw_reg  SystemSampleTime=-1  io_dir=To Processor  arith_type=Unsigned  bitwidth=32  bin_pt=0  sample_period=1  gw_name=ibob_phased_array_2k_xaui_1_rx_linkdown_user_data_in
      link override convert: arith_type=Unsigned  n_bits=32  bin_pt=0
  wires:
  go/1 -> Expression1/2
  din/1 -> XAUI_1/3
  Expression1/1 -> XAUI_1/5
  sync_in/1 -> XAUI_1/4
  Inverter/1 -> Expression1/1
  [linkdown_0] -> Inverter/1
  Constant25/1 -> XAUI_1/2
  Constant22/1 -> XAUI_1/1
  rx_linkdown/1 -> Terminator9/1
  XAUI_1/7 -> Terminator8/1
  XAUI_1/5 -> [linkdown_0], rx_linkdown/1
  XAUI_1/4 -> Terminator6/1
  XAUI_1/3 -> Terminator2/1
  XAUI_1/2 -> Terminator/1
  XAUI_1/1 -> Terminator1/1
  XAUI_1/6 -> Terminator3/1

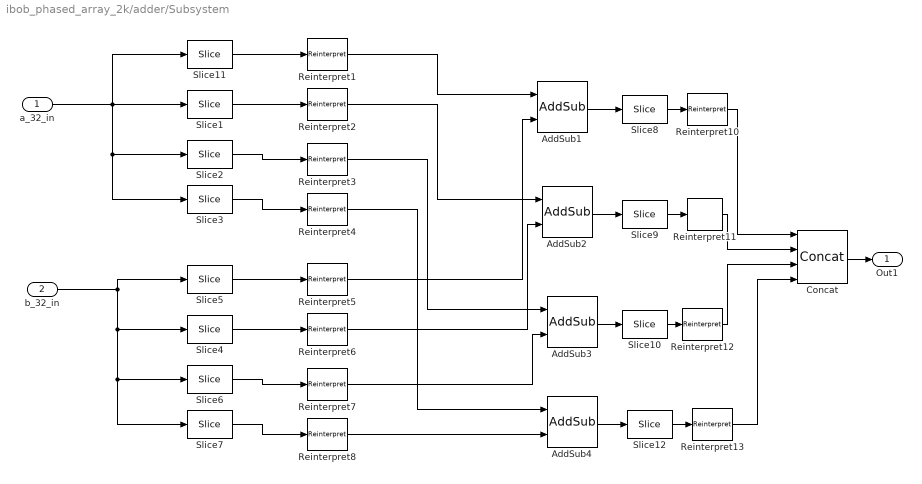
== system ibob_phased_array_2k/adder/Subsystem ==
  a_32_in : Inport  OutDataType=sfix(16)  OutScaling=2^0
  b_32_in : Inport  Port=2  OutDataType=sfix(16)  OutScaling=2^0
  AddSub{1..4} (4 alike) : xbsIndex_r4/AddSub  mode=Addition  use_carryin=off  use_carryout=off  en=off  latency=5  precision=User Defined  arith_type="Signed  (2's comp)"  n_bits=9  bin_pt=6  quantization=Truncate  overflow=Wrap  dbl_ovrd=off  use_behavioral_HDL=on  pipelined=on  use_rpm=on  hw_selection=Fabric  block_type=addsub
      settings: xl_area=[0, 0, 0, 0, 0, 0, 0]  block_version=10.1.3
  Concat : xbsIndex_r4/Concat  num_inputs=4  dbl_ovrd=off  block_type=concat
      settings: block_version=10.1.3
  Reinterpret{1..8} (8 alike) : xbsIndex_r4/Reinterpret  force_arith_type=on  arith_type="Signed  (2's comp)"  force_bin_pt=on  bin_pt=6  block_type=reinterpret
      settings: infoedit="Changes signal type without altering the binary representation.   You can changed the signal between signed and unsigned, and relocate the binary point.<P><P>Hardware notes: In hardware this block costs nothing.<P><P>Example:  Suppose the input is 6 bits wide, signed, with 2 fractional bits, and the output is forced to unsigned with 0 fractional bits.  Then an input of -2.0 (1110.00 in binary 2's complement) becomes an output of 56 (111000 in binary)."  block_version=10.1.3
  Reinterpret{10..13} (4 alike) : xbsIndex_r4/Reinterpret  force_arith_type=on  arith_type=Unsigned  force_bin_pt=on  bin_pt=0  block_type=reinterpret
      settings: infoedit="Changes signal type without altering the binary representation.   You can changed the signal between signed and unsigned, and relocate the binary point.<P><P>Hardware notes: In hardware this block costs nothing.<P><P>Example:  Suppose the input is 6 bits wide, signed, with 2 fractional bits, and the output is forced to unsigned with 0 fractional bits.  Then an input of -2.0 (1110.00 in binary 2's complement) becomes an output of 56 (111000 in binary)."  block_version=10.1.3
  Slice1 : xbsIndex_r4/Slice  nbits=1  boolean_output=off  mode=Two Bit Locations  bit1=23  base1=LSB of Input  bit0=16  base0=LSB of Input  dbl_ovrd=off  block_type=slice
      settings: infoedit="Extracts a given range of bits from each input sample and presents it at the output.  The output type is ordinarily unsigned with binary point at zero, but can be Boolean when the slice is one bit wide.<P><P>Hardware notes: In hardware this block costs nothing."  block_version=10.1.3
  Slice{8..10,12} (4 alike) : xbsIndex_r4/Slice  nbits=1  boolean_output=off  mode=Two Bit Locations  bit1=8  base1=LSB of Input  bit0=1  base0=LSB of Input  dbl_ovrd=off  block_type=slice
      settings: infoedit="Extracts a given range of bits from each input sample and presents it at the output.  The output type is ordinarily unsigned with binary point at zero, but can be Boolean when the slice is one bit wide.<P><P>Hardware notes: In hardware this block costs nothing."  block_version=10.1.3
  Slice11 : xbsIndex_r4/Slice  nbits=1  boolean_output=off  mode=Two Bit Locations  bit1=31  base1=LSB of Input  bit0=24  base0=LSB of Input  dbl_ovrd=off  block_type=slice
      settings: infoedit="Extracts a given range of bits from each input sample and presents it at the output.  The output type is ordinarily unsigned with binary point at zero, but can be Boolean when the slice is one bit wide.<P><P>Hardware notes: In hardware this block costs nothing."  block_version=10.1.3
  Slice2 : xbsIndex_r4/Slice  nbits=1  boolean_output=off  mode=Two Bit Locations  bit1=15  base1=LSB of Input  bit0=8  base0=LSB of Input  dbl_ovrd=off  block_type=slice
      settings: infoedit="Extracts a given range of bits from each input sample and presents it at the output.  The output type is ordinarily unsigned with binary point at zero, but can be Boolean when the slice is one bit wide.<P><P>Hardware notes: In hardware this block costs nothing."  block_version=10.1.3
  Slice3 : xbsIndex_r4/Slice  nbits=1  boolean_output=off  mode=Two Bit Locations  bit1=7  base1=LSB of Input  bit0=0  base0=LSB of Input  dbl_ovrd=off  block_type=slice
      settings: infoedit="Extracts a given range of bits from each input sample and presents it at the output.  The output type is ordinarily unsigned with binary point at zero, but can be Boolean when the slice is one bit wide.<P><P>Hardware notes: In hardware this block costs nothing."  block_version=10.1.3
  Slice4 : xbsIndex_r4/Slice  nbits=1  boolean_output=off  mode=Two Bit Locations  bit1=23  base1=LSB of Input  bit0=16  base0=LSB of Input  dbl_ovrd=off  block_type=slice
      settings: infoedit="Extracts a given range of bits from each input sample and presents it at the output.  The output type is ordinarily unsigned with binary point at zero, but can be Boolean when the slice is one bit wide.<P><P>Hardware notes: In hardware this block costs nothing."  block_version=10.1.3
  Slice5 : xbsIndex_r4/Slice  nbits=1  boolean_output=off  mode=Two Bit Locations  bit1=31  base1=LSB of Input  bit0=24  base0=LSB of Input  dbl_ovrd=off  block_type=slice
      settings: infoedit="Extracts a given range of bits from each input sample and presents it at the output.  The output type is ordinarily unsigned with binary point at zero, but can be Boolean when the slice is one bit wide.<P><P>Hardware notes: In hardware this block costs nothing."  block_version=10.1.3
  Slice6 : xbsIndex_r4/Slice  nbits=1  boolean_output=off  mode=Two Bit Locations  bit1=15  base1=LSB of Input  bit0=8  base0=LSB of Input  dbl_ovrd=off  block_type=slice
      settings: infoedit="Extracts a given range of bits from each input sample and presents it at the output.  The output type is ordinarily unsigned with binary point at zero, but can be Boolean when the slice is one bit wide.<P><P>Hardware notes: In hardware this block costs nothing."  block_version=10.1.3
  Slice7 : xbsIndex_r4/Slice  nbits=1  boolean_output=off  mode=Two Bit Locations  bit1=7  base1=LSB of Input  bit0=0  base0=LSB of Input  dbl_ovrd=off  block_type=slice
      settings: infoedit="Extracts a given range of bits from each input sample and presents it at the output.  The output type is ordinarily unsigned with binary point at zero, but can be Boolean when the slice is one bit wide.<P><P>Hardware notes: In hardware this block costs nothing."  block_version=10.1.3
  Out1 : Outport  OutDataType=sfix(16)  OutScaling=2^0
  wires:
  Concat/1 -> Out1/1
  Reinterpret13/1 -> Concat/4
  Reinterpret12/1 -> Concat/3
  Reinterpret11/1 -> Concat/2
  Reinterpret10/1 -> Concat/1
  Slice12/1 -> Reinterpret13/1
  Slice10/1 -> Reinterpret12/1
  Slice9/1 -> Reinterpret11/1
  Slice8/1 -> Reinterpret10/1
  AddSub4/1 -> Slice12/1
  AddSub3/1 -> Slice10/1
  AddSub2/1 -> Slice9/1
  AddSub1/1 -> Slice8/1
  Reinterpret8/1 -> AddSub4/2
  Reinterpret7/1 -> AddSub3/2
  Reinterpret6/1 -> AddSub2/2
  Reinterpret5/1 -> AddSub1/2
  Reinterpret4/1 -> AddSub4/1
  Reinterpret3/1 -> AddSub3/1
  Reinterpret2/1 -> AddSub2/1
  Reinterpret1/1 -> AddSub1/1
  Slice7/1 -> Reinterpret8/1
  Slice6/1 -> Reinterpret7/1
  Slice4/1 -> Reinterpret6/1
  Slice5/1 -> Reinterpret5/1
  Slice3/1 -> Reinterpret4/1
  Slice2/1 -> Reinterpret3/1
  Slice1/1 -> Reinterpret2/1
  Slice11/1 -> Reinterpret1/1
  b_32_in/1 -> Slice7/1, Slice6/1, Slice4/1, Slice5/1
  a_32_in/1 -> Slice3/1, Slice2/1, Slice1/1, Slice11/1
